simulink model "step3"  (R2020b)
settings: Solver=VariableStepAuto  StartTime=0.0  StopTime=10.0  RelTol=1e-3
libraries: dspadpt3 x2, dspsnks4 x1, dspsrcs4 x1
settings Model: Creator=berkt  LastModifiedBy=berkt

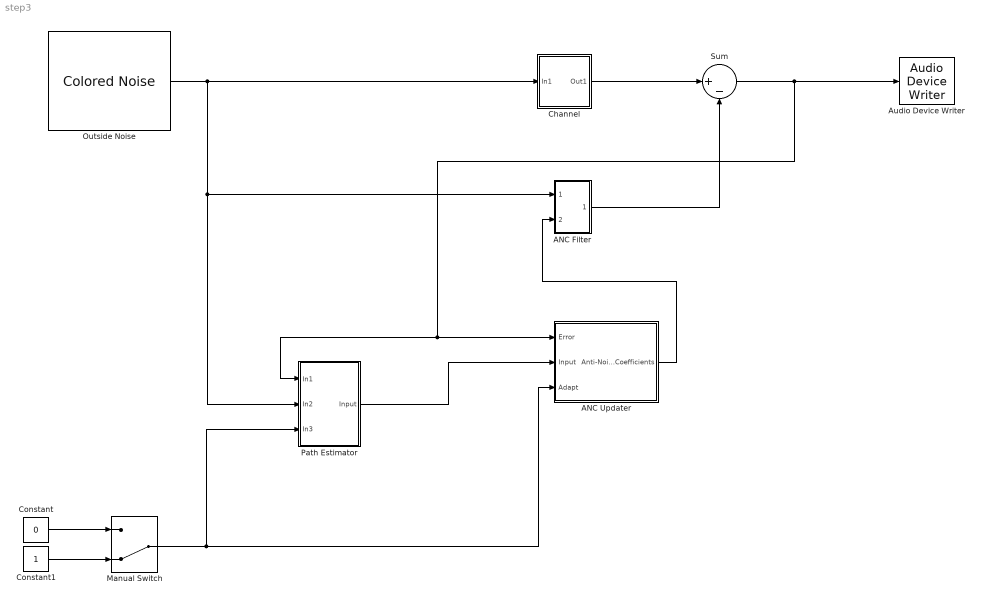
== system step3 ==
  ANC Filter : Subsystem
  ANC Updater : Subsystem
  Audio Device Writer : dspsnks4/Audio Device Writer  Driver=DirectSound  Device=Default  InheritSampleRate=on  SampleRate=44100  BitDepth=16-bit integer  BufferSize=4096  NumBuffers=10  DefaultOutputChannelMapping=on  OutputChannelMapping=1:2  OutputNumUnderrunSamples=off  DriverIdx=1  DeviceWarnFlag=''
  Channel : Subsystem
  Constant : Constant  Value=0
  Constant1 : Constant
  Manual Switch : ManualSwitch  CurrentSetting=0
  Outside Noise : dspsrcs4/Colored Noise  Color=pink  InverseFrequencyPower=1  BoundedOutput=on  NumChannels=1  OutputDataType=double  SamplesPerFrame=1  SampleTime=1/4000  RandomStream=mt19937ar with seed  Seed=67  SimulateUsing=Interpreted execution
      settings: SourceProductName=DSP System Toolbox
  Path Estimator : Subsystem
  Sum : Sum  Inputs=|+-
  wires:
  Outside Noise/1 -> Channel/1(In1), ANC Filter/1(In1), Path Estimator/2(In2)
  Sum/1 -> ANC Updater/1(Error), Path Estimator/1(In1), Audio Device Writer/1
  ANC Filter/1(Out1) -> Sum/2
  ANC Updater/1(Anti-Noise Coefficients) -> ANC Filter/2(In2)
  Channel/1(Out1) -> Sum/1
  Constant/1 -> Manual Switch/1
  Constant1/1 -> Manual Switch/2
  Manual Switch/1 -> ANC Updater/3(Adapt), Path Estimator/3(In3)
  Path Estimator/1(Input) -> ANC Updater/2(Input)

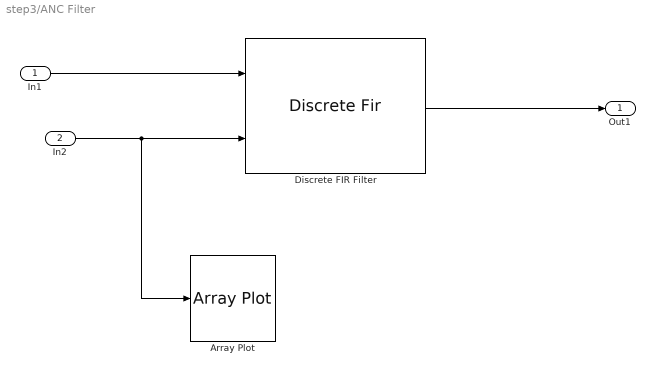
== system step3/ANC Filter ==
  In1 : Inport
  In2 : Inport  Port=2
  Array Plot : ArrayPlot
  Discrete FIR Filter : DiscreteFir  CoefSource=Input port  InputProcessing=Columns as channels (frame based)
      settings: InputPortMap=u0,u1
  Out1 : Outport
  wires:
  In2/1 -> Array Plot/1, Discrete FIR Filter/2
  In1/1 -> Discrete FIR Filter/1
  Discrete FIR Filter/1 -> Out1/1

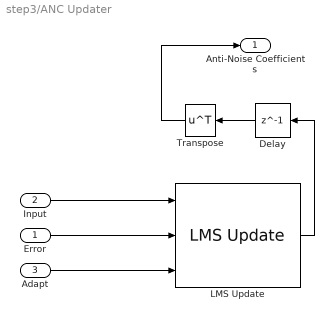
== system step3/ANC Updater ==
  Error : Inport
  Input : Inport  Port=2
  Adapt : Inport  Port=3
  Delay : Delay  DelayLength=1  InitialCondition=0
  LMS Update : dspadpt3/LMS Update  Method=Normalized LMS  Length=32  StepSizeSource=Property  StepSize=0.05  LeakageFactor=1.0  InitialConditions=0  EnableAdaptInput=on  EnableResetInput=off  SimulateUsing=Code generation
      settings: SourceProductBaseCode=DS
  Transpose : Math  Operator=transpose  SaturateOnIntegerOverflow=on
  Anti-Noise Coefficients : Outport
  wires:
  Error/1 -> LMS Update/2
  Delay/1 -> Transpose/1
  Input/1 -> LMS Update/1
  Transpose/1 -> Anti-Noise Coefficients/1
  LMS Update/1 -> Delay/1
  Adapt/1 -> LMS Update/3

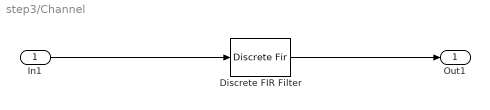
== system step3/Channel ==
  In1 : Inport
  Discrete FIR Filter : DiscreteFir  Coefficients=[0.5 1 -0.3 0.3 0.5 -1 -0.8]  InputProcessing=Columns as channels (frame based)
  Out1 : Outport
  wires:
  Discrete FIR Filter/1 -> Out1/1
  In1/1 -> Discrete FIR Filter/1

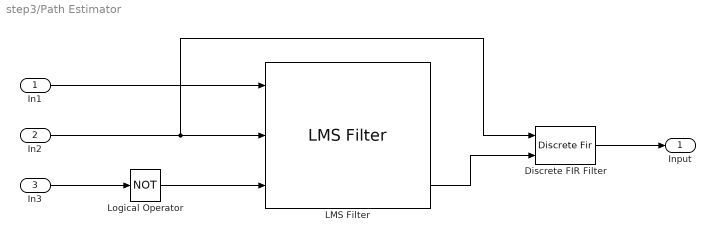
== system step3/Path Estimator ==
  In1 : Inport
  In2 : Inport  Port=2
  In3 : Inport  Port=3
  Discrete FIR Filter : DiscreteFir  CoefSource=Input port  InputProcessing=Columns as channels (frame based)
      settings: InputPortMap=u0,u1
  LMS Filter : dspadpt3/LMS Filter  Algo=Normalized LMS  L=32  stepflag=Dialog  mu=0.05  leakage=1.0  ic=0  Adapt=on  resetflag=None  weights=on  addnparflag=off  roundingMode=Floor  overflowMode=off  secondCoeffMode=Binary point scaling  secondCoeffWordLength=2  secondCoeffFracLength=15  prodOutput2Mode=Binary point scaling  prodOutput2FracLength=20  prodOutput3Mode=Binary point scaling  prodOutput3FracLength=20  prodOutput4Mode=Binary point scaling  prodOutput4FracLength=20  quotientMode=Binary point scaling  quotientFracLength=20  accum2Mode=Binary point scaling  accum2FracLength=20
      settings: SourceProductName=DSP System Toolbox
  Logical Operator : Logic  Operator=NOT  AllPortsSameDT=off  OutDataTypeStr=boolean
  Input : Outport
  wires:
  Discrete FIR Filter/1 -> Input/1
  LMS Filter/3 -> Discrete FIR Filter/2
  In2/1 -> Discrete FIR Filter/1, LMS Filter/2
  In1/1 -> LMS Filter/1
  In3/1 -> Logical Operator/1
  Logical Operator/1 -> LMS Filter/3
